simulink model "like_a_star_1"  (R2020a)
settings: Solver=ode15s  StartTime=0.0  StopTime=400  FixedStep=0.0000001  RelTol=1e-3
values from neighbouring files (symbols this model uses):
  Cwy1 = 0.0074    [Parameters.m]
  Cwy2 = 0.0527    [Parameters.m]
  Cx = 52.92    [Parameters.m]
  Jyy = 0.78    [Parameters.m]
  k1_k = 0.3    [Parameters.m]
  k2_k = 0.16732    [Parameters.m]
  k2_m = 2.19    [Parameters.m]
  K_thruster = 2.89    [Parameters.m]
  kc = 57.2958    [Parameters.m]
  L = 1.760    (= 1.76)    [Parameters.m]
  lambda11 = 0.6    [Parameters.m]
  lambda55 = 0.9    [Parameters.m]
  m = 24.7    [Parameters.m]
  Rmin = 0.4    [Parameters.m]
  T_thruster = 0.1    [Parameters.m]
  Vz = 0    [Parameters.m]
libraries: simulink x6, simulink_extras x1
settings Model: EnablePacing=on  PacingRate=0.500000  Creator=Eugene  LastModifiedBy=corsair
settings DataIOCC: ReturnWorkspaceOutputs=off
settings DebuggingCC: ParameterOverflowMsg=warning  ArithmeticOperatorsInVariantConditions=warning
settings HardwareCC: ProdHWDeviceType=AMD->x86-64 (Windows64)
settings SFSimCC: SimUseLocalCustomCode=off  CustomCodeUndefinedFunction=UseInterfaceOnly
settings RTWCC: RTWUseLocalCustomCode=off

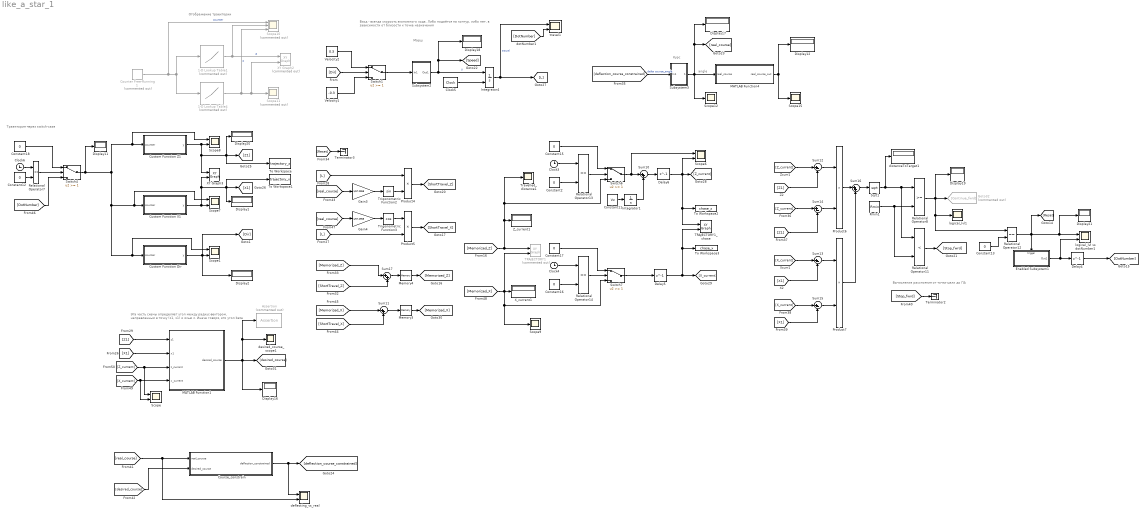
== system like_a_star_1 ==
  note: Траектория через switch-case
  note: Вход - всегда скорость экономного хода. Либо подаётся на контур, либо нет, в зависимости от близости к точке назначения
  note: Курс
  note: Отображение траектории
  note: Марш
  note: Вычисление расстояния от точки-цели до ПА
  note: Эта часть схемы определяет угол между радиус-вектором, направленным в точку (z1, x1) и осью z. Иначе говоря, это угол beta
  note: angle
  1-D Lookup Table1 : Lookup_n-D  Commented=on  NumberOfTableDimensions=1  BreakpointsForDimension1=[0:7]  BreakpointsForDimension1FirstPoint=0  BreakpointsForDimension1DataTypeStr=uint8  Table=[0,0,L,L,2*L,2*L,3*L, 3*L]  TableDataTypeStr=double  InterpMethod=Flat  ExtrapMethod=Cubic spline  RemoveProtectionInput=on  InternalRulePriority=Speed  OutDataTypeStr=double  RndMeth=Zero  InputSameDT=on
  1-D Lookup Table4 : Lookup_n-D  Commented=on  NumberOfTableDimensions=1  BreakpointsForDimension1=[0:7]  BreakpointsForDimension1DataTypeStr=int16  Table=[0,25,25,0,0,25,25,0]  TableDataTypeStr=double  InterpMethod=Flat  RemoveProtectionInput=on  InternalRulePriority=Speed  OutDataTypeStr=double  RndMeth=Zero  InputSameDT=on
  Assertion : Assertion  Commented=on  AssertionFailFcn=-1
  Clock3 : Clock
  Clock4 : Clock
  Clock5 : simulink_extras/Flip Flops/Clock  period=0.05
  Clock6 : Clock
  Constant11 : Constant  Value=Vz
  Constant{2,12..13,15..18} (7 alike) : Constant  Value=0
  Counter Free-Running1 : simulink/Sources/Counter Free-Running  Commented=on  NumBits=3  tsamp=1
  Course_constrain : MATLAB Function  TreatAsAtomicUnit=on
  Custom Function Dir : MATLAB Function  TreatAsAtomicUnit=on
  Custom Function X1 : MATLAB Function  TreatAsAtomicUnit=on
  Custom Function Z1 : MATLAB Function  TreatAsAtomicUnit=on
  Delay4 : Delay  DelayLength=1  InitialCondition=0  SampleTime=0.05
  Delay5 : Delay  DelayLength=1  SampleTime=0.05
  Delay6 : Delay  DelayLength=1  SampleTime=0.05
  Display{1..2,11..12,16..21} (10 alike) : Display
  Enabled Subsystem1 : Subsystem  TreatAsAtomicUnit=on
  Gain3 : Gain  Gain=1/57.2958
  Gain4 : Gain  Gain=1/57.2958
  Goto32 : Goto  Commented=on  GotoTag=Continue_fwrd
  Integrator1 : Integrator
  Integrator4 : Integrator  ExternalReset=rising
  MATLAB Function1 : MATLAB Function  TreatAsAtomicUnit=on
  MATLAB Function4 : MATLAB Function  TreatAsAtomicUnit=on
  Memory3 : Memory  InitialCondition=15
  Memory4 : Memory
  Product{4..7} (4 alike) : Product
  Relational Operator11 : RelationalOperator  Operator=<  OutDataTypeStr=boolean  RndMeth=Simplest
  Relational Operator{7,12..14} (4 alike) : RelationalOperator  Operator===  OutDataTypeStr=boolean  RndMeth=Simplest
  Relational Operator8 : RelationalOperator  OutDataTypeStr=boolean  RndMeth=Simplest
  Rmin1 : Constant  Value=Rmin
  Scope{,1,6..8} (5 alike) : Scope  NumInputPorts=2
  Scope10 : Scope  Commented=on  NumInputPorts=3
  Scope11 : Scope  Commented=on
  Scope12 : Scope
  Scope15 : Scope
  Scope9 : Scope
  Sqrt1 : Sqrt  SaturateOnIntegerOverflow=on
  Subsystem2 : Subsystem
  Subsystem3 : Subsystem
  Sum{10..11,16..17} (4 alike) : Sum  Inputs=|++
  Sum{12..15} (4 alike) : Sum  Inputs=|+-
  Switch{1,4,6..7} (4 alike) : Switch  Threshold=1
  TRAJECTORY1 : simulink/Sinks/XY Graph  Commented=on  xmin=-1  xmax=10  ymin=-5  ymax=30  st=-1
  TRAJECTORY1_chase : simulink/Sinks/XY Graph  xmin=-15  xmax=15  ymin=-15  ymax=15  st=-1
  Terminator2 : Terminator
  Terminator3 : Terminator
  To Workspace : ToWorkspace  VariableName=trajectory_z  SampleTime=-1
  To Workspace1 : ToWorkspace  VariableName=trajectory_x  SampleTime=-1
  To Workspace2 : ToWorkspace  VariableName=chase_z  SampleTime=-1
  To Workspace3 : ToWorkspace  VariableName=chase_x  SampleTime=-1
  Travelled_distance1 : Scope
  Trigonometric Function2 : Trigonometry
  Trigonometric Function3 : Trigonometry  Operator=cos
  Velocity1 : Constant  Value=-0.3
  Velocity2 : Constant  Value=0.3
  XY Graph2 : simulink/Sinks/XY Graph  Commented=on  xmin=-10  xmax=20  ymin=-10  ymax=30  st=-1
  XY Graph3 : simulink/Sinks/XY Graph  xmin=-15  xmax=15  ymin=-15  ymax=15  st=-1
  X_current1 : Display
  Z_current1 : Display
  deflecting_vs_real : Scope  NumInputPorts=2
  desired_course_scope1 : Scope
  distanceToTarget1 : Display
  logical_lvl vs dotNumber1 : Scope  NumInputPorts=2
  logical_lvl1 : Scope
  travel1 : Scope  NumInputPorts=2
  wires:
  Sum11/1 -> Memory3/1
  Switch4/1 -> Scope1/1, Custom Function Dir/1(counter), Custom Function X1/1(counter), Scope7/1, Scope8/1, Custom Function Z1/1(counter), Display11/1
  Sum14/1 -> Product6/2
  [Stop_fwrd] -> Terminator2/1
  1-D Lookup Table1/1 -> XY Graph2/1, Scope10/2  "Z"
  Clock6/1 -> Relational Operator7/1
  Subsystem2/1(Out1) -> [Speed], Display18/1, Integrator4/1  "V"
  Delay6/1 -> TRAJECTORY1_chase/1, To Workspace2/1, [Z_current], Scope6/2
  [Reset] -> Terminator3/1
  Constant18/1 -> Switch4/1
  [DotNumber] -> travel1/2
  [X1] -> MATLAB Function1/2(x1)
  Relational Operator7/1 -> Switch4/2
  [real_course] -> deflecting_vs_real/2, Course_constrain/1(real_course)
  MATLAB Function1/1(desired_course) -> [desired_course], Display16/1, Assertion/1, desired_course_scope1/1
  Course_constrain/1(deflection_constrained) -> deflecting_vs_real/1, [deflection_course_constrained]
  [real_course] -> Gain3/1
  MATLAB Function4/1(real_course_out) -> Scope15/1, Display12/1
  Constant12/1 -> Relational Operator7/2
  Switch6/1 -> Scope6/1, Sum10/1
  Memory3/1 -> [Memorized_X]
  [Z_current] -> MATLAB Function1/3(z_current), Scope/1
  Product4/1 -> [ShortTravel_Z]
  [ShortTravel_X] -> Sum11/2
  Sum17/1 -> Memory4/1
  Sum13/1 -> Product7/1
  Trigonometric Function2/1 -> Product4/2
  [Z1] -> Sum14/2
  [Z_current] -> Sum14/1
  [X1] -> Sum13/2
  [Z_current] -> Sum12/1
  Integrator4/1 -> [L], travel1/1  "travel"
  [L] -> Product4/1
  Gain3/1 -> Trigonometric Function2/1
  Sum12/1 -> Product6/1
  Delay4/1 -> [DotNumber]
  Sum15/1 -> Product7/2
  1-D Lookup Table4/1 -> Scope11/1, XY Graph2/2, Scope10/3  "X"
  Counter Free-Running1/1 -> Scope10/1, 1-D Lookup Table1/1, 1-D Lookup Table4/1  "counter"
  Product7/1 -> Sum16/2
  Constant15/1 -> Switch6/1
  Custom Function Z1/1(y) -> Scope8/2, To Workspace/1, Display20/1, [Z1], XY Graph3/1
  Constant13/1 -> Relational Operator12/2
  Relational Operator12/1 -> [Reset], Enabled Subsystem1/Trigger, logical_lvl vs dotNumber1/1, Display21/1
  [X_current] -> Sum15/1
  Subsystem3/1(Out1) -> [real_course], Display17/1, Scope12/1, MATLAB Function4/1(real_course)
  Relational Operator11/1 -> [Stop_fwrd]
  Integrator1/1 -> Sum10/2
  Rmin1/1 -> Relational Operator8/2, Relational Operator11/2
  [X1] -> Sum15/2
  Sum16/1 -> Sqrt1/1
  [X_current] -> Sum13/1
  [Memorized_Z] -> Sum17/1
  Switch7/1 -> Delay5/1
  [DotNumber] -> Switch4/3
  [X_current] -> Scope/2, MATLAB Function1/4(x_current)
  [Memorized_Z] -> Switch6/3, Travelled_distance1/1, Z_current1/1, TRAJECTORY1/1
  [Z1] -> Sum12/2
  Constant2/1 -> Relational Operator13/2
  Custom Function X1/1(y) -> To Workspace1/1, Display1/1, [X1], XY Graph3/2, Scope7/2
  Product6/1 -> Sum16/1
  [ShortTravel_Z] -> Sum17/2
  [deflection_course_constrained] -> Subsystem3/1(In1)  "delta course_angle"
  Switch1/1 -> Subsystem2/1(In1)
  Clock4/1 -> Relational Operator14/1
  [Z1] -> MATLAB Function1/1(z1)
  Constant17/1 -> Switch7/1
  Relational Operator14/1 -> Switch7/2
  Clock5/1 -> Integrator4/2
  Gain4/1 -> Trigonometric Function3/1
  [L] -> Product5/2
  [desired_course] -> Course_constrain/2(desired_course)
  Sum10/1 -> Delay6/1
  Clock3/1 -> Relational Operator13/1
  Product5/1 -> [ShortTravel_X]
  Delay5/1 -> [X_current], TRAJECTORY1_chase/2, To Workspace3/1
  [Memorized_X] -> Sum11/1
  Enabled Subsystem1/1(Out1) -> Delay4/1, logical_lvl vs dotNumber1/2
  Relational Operator13/1 -> Switch6/2
  [Memorized_X] -> Switch7/3, Scope9/1, TRAJECTORY1/2, X_current1/1
  Trigonometric Function3/1 -> Product5/1
  Relational Operator8/1 -> Display19/1, Relational Operator12/1, logical_lvl1/1, Goto32/1
  Constant16/1 -> Relational Operator14/2
  [real_course] -> Gain4/1
  Memory4/1 -> [Memorized_Z]
  Constant11/1 -> Integrator1/1
  Sqrt1/1 -> Relational Operator8/1, Relational Operator11/1, distanceToTarget1/1
  Custom Function Dir/1(y) -> Display2/1, [Dir], Scope1/2
  [Dir] -> Switch1/2
  Velocity2/1 -> Switch1/1
  Velocity1/1 -> Switch1/3

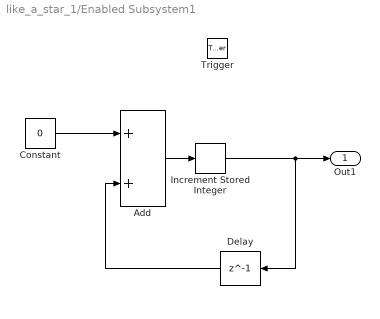
== system like_a_star_1/Enabled Subsystem1 ==
  Trigger : TriggerPort  VariantControl=Variant  PortDimensions=1
  Add : Sum
  Constant : Constant  Value=0
  Delay : Delay  DelayLength=1  InitialCondition=0
  Increment Stored Integer : simulink/Additional Math & Discrete/Additional Math: Increment - Decrement/Increment Stored Integer
  Out1 : Outport  VectorParamsAs1DForOutWhenUnconnected=off
  wires:
  Constant/1 -> Add/1
  Delay/1 -> Add/2
  Add/1 -> Increment Stored Integer/1
  Increment Stored Integer/1 -> Delay/1, Out1/1

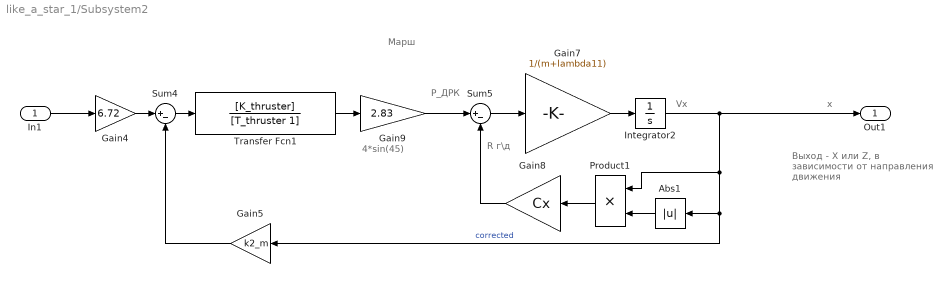
== system like_a_star_1/Subsystem2 ==
  note: Выход - X или Z, в зависимости от направления движения
  note: 4*sin(45)
  note: R г\д
  note: x
  note: Vx
  note: P_ДРК
  note: Марш
  In1 : Inport
  Abs1 : Abs
  Gain4 : Gain  Gain=6.72
  Gain5 : Gain  Gain=k2_m
  Gain7 : Gain  Gain=1/(m+lambda11)
  Gain8 : Gain  Gain=Cx
  Gain9 : Gain  Gain=2.83
  Integrator2 : Integrator  InitialCondition=0.7
  Product1 : Product
  Sum4 : Sum  Inputs=|+-
  Sum5 : Sum  Inputs=|+-
  Transfer Fcn1 : TransferFcn  Numerator=[K_thruster]  Denominator=[T_thruster 1]
  Out1 : Outport  VectorParamsAs1DForOutWhenUnconnected=off
  wires:
  In1/1 -> Gain4/1
  Product1/1 -> Gain8/1
  Gain7/1 -> Integrator2/1
  Gain8/1 -> Sum5/2
  Integrator2/1 -> Out1/1, Gain5/1, Abs1/1, Product1/1  "corrected"
  Transfer Fcn1/1 -> Gain9/1
  Gain4/1 -> Sum4/1
  Sum4/1 -> Transfer Fcn1/1
  Sum5/1 -> Gain7/1
  Gain9/1 -> Sum5/1
  Gain5/1 -> Sum4/2
  Abs1/1 -> Product1/2

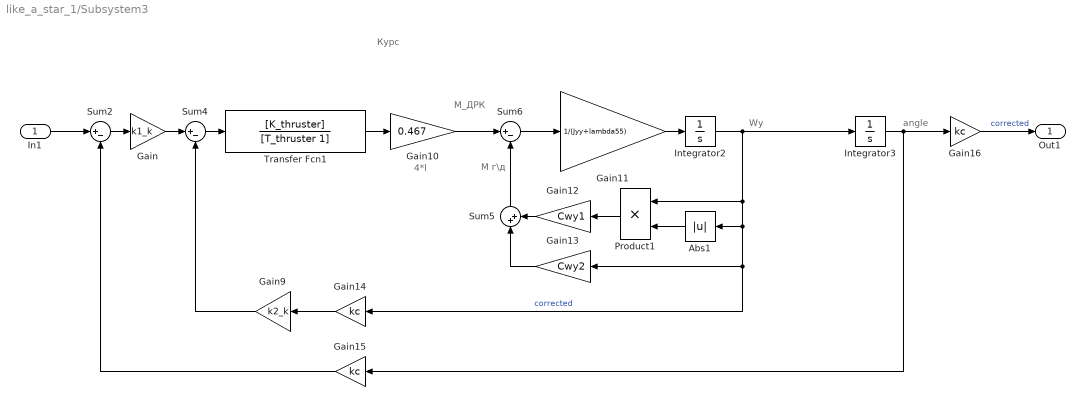
== system like_a_star_1/Subsystem3 ==
  note: Курс
  note: Wy
  note: M_ДРК
  note: 4*l
  note: angle
  note: M г\д
  In1 : Inport
  Abs1 : Abs
  Gain : Gain  Gain=k1_k
  Gain10 : Gain  Gain=0.467
  Gain11 : Gain  Gain=1/(Jyy+lambda55)
  Gain12 : Gain  Gain=Cwy1
  Gain13 : Gain  Gain=Cwy2
  Gain14 : Gain  Gain=kc
  Gain15 : Gain  Gain=kc
  Gain16 : Gain  Gain=kc
  Gain9 : Gain  Gain=k2_k
  Integrator2 : Integrator
  Integrator3 : Integrator  InitialCondition=180
  Product1 : Product
  Sum2 : Sum  Inputs=|+-
  Sum4 : Sum  Inputs=|+-
  Sum5 : Sum  Inputs=|++
  Sum6 : Sum  Inputs=|+-
  Transfer Fcn1 : TransferFcn  Numerator=[K_thruster]  Denominator=[T_thruster 1]
  Out1 : Outport  VectorParamsAs1DForOutWhenUnconnected=off
  wires:
  Gain12/1 -> Sum5/2
  Gain10/1 -> Sum6/1
  Product1/1 -> Gain12/1
  Gain11/1 -> Integrator2/1
  Gain9/1 -> Sum4/2
  Gain/1 -> Sum4/1
  Transfer Fcn1/1 -> Gain10/1
  Sum6/1 -> Gain11/1
  Gain14/1 -> Gain9/1
  Gain15/1 -> Sum2/2
  Gain13/1 -> Sum5/1
  Abs1/1 -> Product1/2
  Sum5/1 -> Sum6/2
  Integrator2/1 -> Gain14/1, Gain13/1, Abs1/1, Product1/1, Integrator3/1  "corrected"
  Sum2/1 -> Gain/1
  Integrator3/1 -> Gain16/1, Gain15/1
  Sum4/1 -> Transfer Fcn1/1
  In1/1 -> Sum2/1
  Gain16/1 -> Out1/1  "corrected"

== matlab function like_a_star_1/Custom Function Dir ==
  data: counter input; y output
function y = fcn(counter)

%L = 1.76;
% 1 - fwd, -1 - backward

    if counter % 2 == 1
        y = 1;
    else
        y = -1;
    end
end

== matlab function like_a_star_1/Custom Function Z1 ==
  data: counter input; y output
function y = fcn( counter)

%L = 1.76;



switch counter
    case 1
      y = 5.75;
    case 2
      y = 12.56;
    case 3
      y = 5.36;
    case 4
      y = 11.26;
    case 5
      y = 4.6;
    case 6
      y = 9.19;
    case 7
      y = 3.53;
     
   otherwise
      y = 13;
end

== matlab function like_a_star_1/Custom Function X1 ==
  data: counter input; y output
function y = fcn(counter)

%L = 1.76;

switch counter
   
    case 1
      y = -0.76;
    case 2
        y = -3.36;
    case 3
      y = -2.22;
    case 4
      y = -6.5;
    case 5
      y = -3.53;
    case 6
      y = -9.19;
    case 7
        y = -4.6;
   otherwise
      y = 0;

end

== matlab function like_a_star_1/MATLAB Function1 ==
  data: z1 input; x1 input; z_current input; desired_course output; x_current input
function desired_course = fcn(z1, x1, z_current, x_current)

delta_x = x1 - x_current;
delta_z = z1 - z_current;

%1
if (delta_x >= 0) && (delta_z >= 0)
    desired_course = 57.2958*atan(delta_z / delta_x);
%2    
elseif (delta_x >= 0) && (delta_z < 0)
    desired_course = 360 - 57.2958*atan( abs(delta_z) / delta_x);
%3    
elseif (delta_x < 0) && (delta_z < 0)    
    desired_course = 180 + 57.2958*atan(abs(delta_z) / abs(delta_x));
%4    
elseif (delta_x < 0) && (delta_z >= 0)    
    desired_course = 180 - 57.2958*atan( delta_z / abs(delta_x));   
    
else 
    desired_course = -1;
   
end

== matlab function like_a_star_1/MATLAB Function4 ==
  data: real_course input; real_course_out output
function real_course_out   = fcn(real_course)

    % Приводим к стандарту
    if real_course < 0
        real_course_out = 360 - abs(real_course);
    elseif real_course >= 360
        real_course_out = real_course - 360;
    else    
        real_course_out = real_course;
    end

end

== matlab function like_a_star_1/Course_constrain ==
  data: real_course input; desired_course input; deflection_constrained output
function deflection_constrained   = fcn(real_course, desired_course)

    % предстоит повернуться более чем на 180 градусов
    % текущее положение курса не имеет никакого значения,
    %важно лишь конечное положение.
    % Па должен поворачиват менее чем на 180 градусов
    
    if abs(desired_course - real_course) > 180
    % выполняем ограничение
        if desired_course > 180
            deflection_constrained = desired_course - 360;
        %elseif desired_course < -180
        %    deflection_constrained = 360 + desired_course;
        else
            deflection_constrained = desired_course;
        end
    % иначе просто приравниваем
    else
        deflection_constrained = desired_course;
    end
end
